simulink model "RedCrane_kinematic_model_joystic"  (R2024a)
settings: Solver=FixedStepAuto  StartTime=0.0  StopTime=inf  FixedStep=Ts  MaxStep=0.005  RelTol=1e-3
values from neighbouring files (symbols this model uses):
  Cartesian_home = [3.55, 0.4, 1.6]'    [enviroment_setup.m]
  M = [1, 0, 0, (L5 + L4 - L1) ... (first row only)    [enviroment_setup.m]
  SList = [ws_mat ... (first row only)    [enviroment_setup.m]
  telescope0 = 0    [enviroment_setup.m]
  thetaList0 = [0, 0,-pi/8, 0, 0]'    [enviroment_setup.m]
  Ts = 0.001    [enviroment_setup.m]
undefined symbols (not defined in the file or in its folder): dp_k_angle_to_stroke, dp_m_angle_to_stroke, p_k_angle_to_stroke, p_k_stroke_to_angle, p_m_angle_to_stroke, p_m_stroke_to_angle, X, Y, Z
libraries: sm_lib x82, nesl_utility x19, fl_lib x16, TcSimInterface x2
(part 3 of 3)

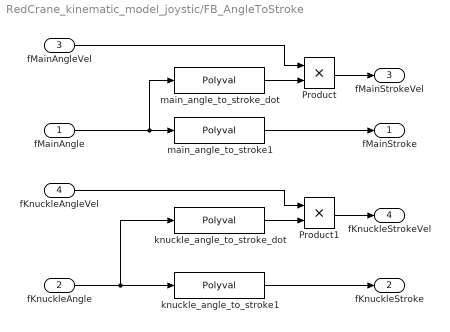
== system RedCrane_kinematic_model_joystic/FB_AngleToStroke ==
  fMainAngle : Inport
  fKnuckleAngle : Inport  Port=2
  fMainAngleVel : Inport  Port=3
  fKnuckleAngleVel : Inport  Port=4
  Product : Product
  Product1 : Product
  knuckle_angle_to_stroke1 : Polyval  Coefs=p_k_angle_to_stroke
  knuckle_angle_to_stroke_dot : Polyval  Coefs=dp_k_angle_to_stroke
  main_angle_to_stroke1 : Polyval  Coefs=p_m_angle_to_stroke
  main_angle_to_stroke_dot : Polyval  Coefs=dp_m_angle_to_stroke
  fMainStroke : Outport
  fKnuckleStroke : Outport  Port=2
  fMainStrokeVel : Outport  Port=3
  fKnuckleStrokeVel : Outport  Port=4
  wires:
  fMainAngle/1 -> main_angle_to_stroke_dot/1, main_angle_to_stroke1/1
  knuckle_angle_to_stroke_dot/1 -> Product1/2
  fKnuckleAngleVel/1 -> Product1/1
  fKnuckleAngle/1 -> knuckle_angle_to_stroke_dot/1, knuckle_angle_to_stroke1/1
  knuckle_angle_to_stroke1/1 -> fKnuckleStroke/1
  main_angle_to_stroke_dot/1 -> Product/2
  main_angle_to_stroke1/1 -> fMainStroke/1
  Product1/1 -> fKnuckleStrokeVel/1
  Product/1 -> fMainStrokeVel/1
  fMainAngleVel/1 -> Product/1

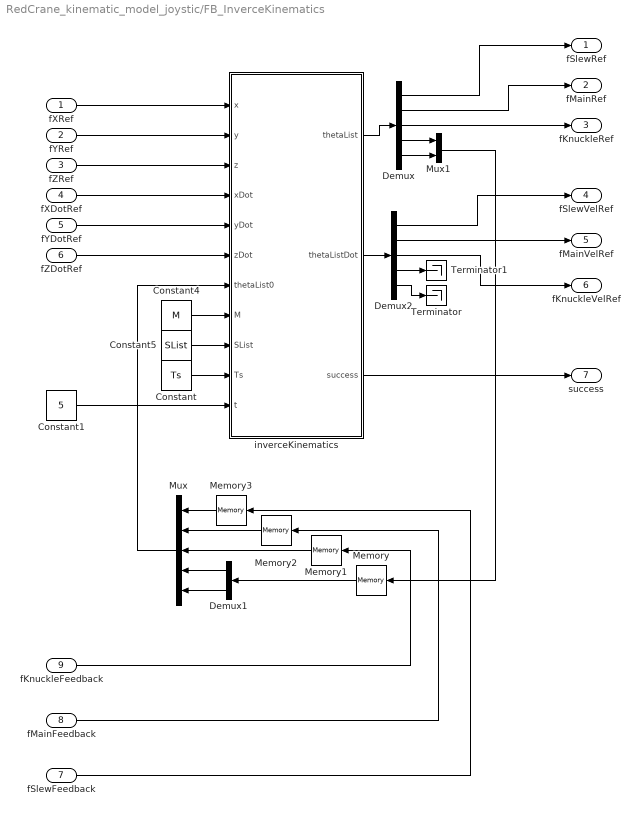
== system RedCrane_kinematic_model_joystic/FB_InverceKinematics ==
  fXRef : Inport
  fYRef : Inport  Port=2
  fZRef : Inport  Port=3
  fXDotRef : Inport  Port=4
  fYDotRef : Inport  Port=5
  fZDotRef : Inport  Port=6
  fSlewFeedback : Inport  Port=7
  fMainFeedback : Inport  Port=8
  fKnuckleFeedback : Inport  Port=9
  Constant : Constant  Value=Ts
  Constant1 : Constant  Value=5
  Constant4 : Constant  Value=M
  Constant5 : Constant  Value=SList
  Demux : Demux  Outputs=5
  Demux1 : Demux  Outputs=2
  Demux2 : Demux  Outputs=5
  Memory : Memory  InitialCondition=[thetaList0(4), thetaList0(5)]'
  Memory1 : Memory  InitialCondition=thetaList0(3)
  Memory2 : Memory  InitialCondition=thetaList0(2)
  Memory3 : Memory  InitialCondition=thetaList0(1)
  Mux : Mux  Inputs=5
  Mux1 : Mux  Inputs=2
  Terminator : Terminator
  Terminator1 : Terminator
  inverceKinematics : MATLAB Function  TreatAsAtomicUnit=on
  fSlewRef : Outport
  fMainRef : Outport  Port=2
  fKnuckleRef : Outport  Port=3
  fSlewVelRef : Outport  Port=4
  fMainVelRef : Outport  Port=5
  fKnuckleVelRef : Outport  Port=6
  success : Outport  Port=7
  wires:
  Memory1/1 -> Mux/3
  Demux/5 -> Mux1/2
  Constant4/1 -> inverceKinematics/8(M)
  Memory3/1 -> Mux/1
  Demux2/5 -> Terminator/1
  fSlewFeedback/1 -> Memory3/1
  Demux1/2 -> Mux/5
  Memory2/1 -> Mux/2
  Constant5/1 -> inverceKinematics/9(SList)
  Demux2/1 -> fSlewVelRef/1
  fXDotRef/1 -> inverceKinematics/4(xDot)
  inverceKinematics/1(thetaList) -> Demux/1
  Constant1/1 -> inverceKinematics/11(t)
  Demux/1 -> fSlewRef/1
  fXRef/1 -> inverceKinematics/1(x)
  Constant/1 -> inverceKinematics/10(Ts)
  Demux1/1 -> Mux/4
  Mux/1 -> inverceKinematics/7(thetaList0)
  Mux1/1 -> Memory/1
  fZRef/1 -> inverceKinematics/3(z)
  Memory/1 -> Demux1/1
  inverceKinematics/2(thetaListDot) -> Demux2/1
  Demux/4 -> Mux1/1
  Demux2/4 -> Terminator1/1
  fMainFeedback/1 -> Memory2/1
  fYRef/1 -> inverceKinematics/2(y)
  fKnuckleFeedback/1 -> Memory1/1
  Demux/3 -> fKnuckleRef/1
  fYDotRef/1 -> inverceKinematics/5(yDot)
  fZDotRef/1 -> inverceKinematics/6(zDot)
  Demux2/3 -> fKnuckleVelRef/1
  Demux/2 -> fMainRef/1
  Demux2/2 -> fMainVelRef/1
  inverceKinematics/3(success) -> success/1

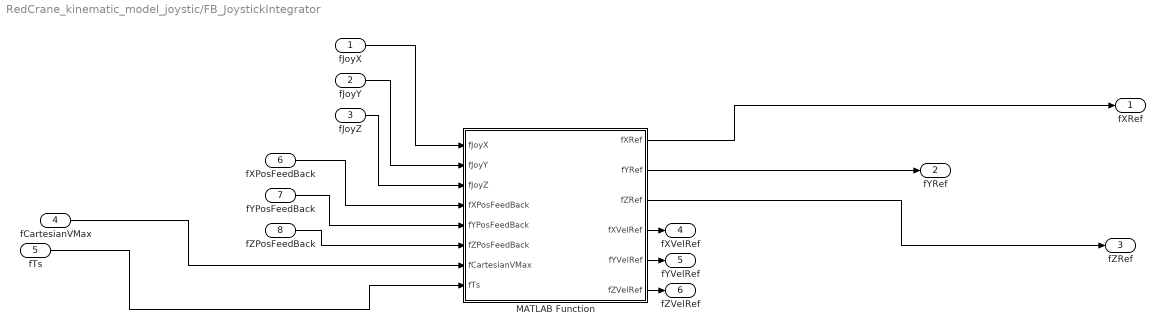
== system RedCrane_kinematic_model_joystic/FB_JoystickIntegrator ==
  fJoyX : Inport
  fJoyY : Inport  Port=2
  fJoyZ : Inport  Port=3
  fCartesianVMax : Inport  Port=4
  fTs : Inport  Port=5
  fXPosFeedBack : Inport  Port=6
  fYPosFeedBack : Inport  Port=7
  fZPosFeedBack : Inport  Port=8
  MATLAB Function : MATLAB Function  TreatAsAtomicUnit=on
  fXRef : Outport
  fYRef : Outport  Port=2
  fZRef : Outport  Port=3
  fXVelRef : Outport  Port=4
  fYVelRef : Outport  Port=5
  fZVelRef : Outport  Port=6
  wires:
  fJoyY/1 -> MATLAB Function/2(fJoyY)
  fCartesianVMax/1 -> MATLAB Function/7(fCartesianVMax)
  MATLAB Function/6(fZVelRef) -> fZVelRef/1
  MATLAB Function/4(fXVelRef) -> fXVelRef/1
  MATLAB Function/5(fYVelRef) -> fYVelRef/1
  fTs/1 -> MATLAB Function/8(fTs)
  fJoyX/1 -> MATLAB Function/1(fJoyX)
  fJoyZ/1 -> MATLAB Function/3(fJoyZ)
  fXPosFeedBack/1 -> MATLAB Function/4(fXPosFeedBack)
  fYPosFeedBack/1 -> MATLAB Function/5(fYPosFeedBack)
  fZPosFeedBack/1 -> MATLAB Function/6(fZPosFeedBack)
  MATLAB Function/2(fYRef) -> fYRef/1
  MATLAB Function/1(fXRef) -> fXRef/1
  MATLAB Function/3(fZRef) -> fZRef/1

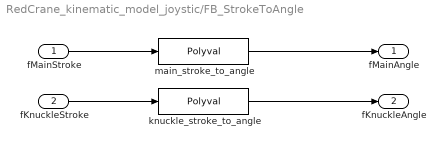
== system RedCrane_kinematic_model_joystic/FB_StrokeToAngle ==
  fMainStroke : Inport
  fKnuckleStroke : Inport  Port=2
  knuckle_stroke_to_angle : Polyval  Coefs=p_k_stroke_to_angle
  main_stroke_to_angle : Polyval  Coefs=p_m_stroke_to_angle
  fMainAngle : Outport
  fKnuckleAngle : Outport  Port=2
  wires:
  fKnuckleStroke/1 -> knuckle_stroke_to_angle/1
  fMainStroke/1 -> main_stroke_to_angle/1
  main_stroke_to_angle/1 -> fMainAngle/1
  knuckle_stroke_to_angle/1 -> fKnuckleAngle/1

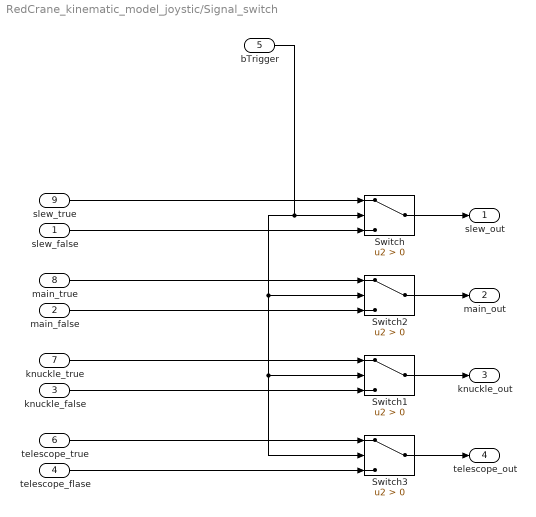
== system RedCrane_kinematic_model_joystic/Signal_switch ==
  slew_false : Inport
  main_false : Inport  Port=2
  knuckle_false : Inport  Port=3
  telescope_flase : Inport  Port=4
  bTrigger : Inport  Port=5
  telescope_true : Inport  Port=6
  knuckle_true : Inport  Port=7
  main_true : Inport  Port=8
  slew_true : Inport  Port=9
  Switch{,1..3} (4 alike) : Switch  Criteria=u2 > Threshold  SaturateOnIntegerOverflow=off  InputSameDT=off
  slew_out : Outport
  main_out : Outport  Port=2
  knuckle_out : Outport  Port=3
  telescope_out : Outport  Port=4
  wires:
  Switch1/1 -> knuckle_out/1
  bTrigger/1 -> Switch2/2, Switch1/2, Switch3/2, Switch/2
  telescope_true/1 -> Switch3/1
  slew_false/1 -> Switch/3
  Switch2/1 -> main_out/1
  slew_true/1 -> Switch/1
  knuckle_true/1 -> Switch1/1
  Switch3/1 -> telescope_out/1
  main_false/1 -> Switch2/3
  Switch/1 -> slew_out/1
  telescope_flase/1 -> Switch3/3
  knuckle_false/1 -> Switch1/3
  main_true/1 -> Switch2/1

== matlab function RedCrane_kinematic_model_joystic/FB_InverceKinematics/inverceKinematics ==
  data: x input; thetaList output size=[5, 1]; y input; z input; xDot input; yDot input; zDot input; thetaList0 input; M input; SList input; Ts input; thetaListDot output size=[5, 1]; success output size=1; t input
function [thetaList, thetaListDot, success] = inverceKinematics( ...
    x, y, z, xDot, yDot, zDot, thetaList0, M, SList, Ts, t)

if(t <= Ts*1.1)
    thetaList0 = [0, 0, 0, 0, 0]';
end

% Explicitly pre-assign outputs
thetaList    = zeros(5,1);
thetaListDot = zeros(5,1);
success      = false;    % or 0 if you prefer numeric


T = [1 0 0 x;
    0 1 0 y;
    0 0 1 z;
    0 0 0 1];


[thetaOut, successOut] = IKinSpace(SList, M, T, thetaList0, 0.00001, 0.0000001);

% Assign them to the pre-allocated outputs
thetaList    = thetaOut;
success      = successOut;


Js = JacobianSpace(SList,thetaList);
Js_pinv = pinv(Js);
xyzDot = [0;
         0;
         0;
         xDot;
         yDot;
         zDot
         ];

thetaListDot = Js_pinv*xyzDot;

end

== matlab function RedCrane_kinematic_model_joystic/FB_JoystickIntegrator/MATLAB Function ==
  data: fJoyX input; fJoyY input; fJoyZ input; fXPosFeedBack input; fXRef output; fYRef output; fZRef output; fXVelRef output; fYVelRef output; fZVelRef output; fYPosFeedBack input; fZPosFeedBack input; fCartesianVMax input; fTs input
function [fXRef, fYRef, fZRef, fXVelRef, fYVelRef, fZVelRef]  = fcn(fJoyX, fJoyY, fJoyZ, fXPosFeedBack, fYPosFeedBack, fZPosFeedBack, fCartesianVMax, fTs)

fXVelRef = fCartesianVMax*fJoyX;
fYVelRef = fCartesianVMax*fJoyY;
fZVelRef = fCartesianVMax*fJoyZ;

fXRef = fXPosFeedBack + fXVelRef*fTs;
fYRef = fYPosFeedBack + fYVelRef*fTs; 
fZRef = fZPosFeedBack + fZVelRef*fTs;
